simulink subsystem "Accelerometer"  (R2024b)
settings: Solver=VariableStepAuto  StartTime=0.0  StopTime=10.0  RelTol=1e-3
values from neighbouring files (symbols this model uses):
  g = 9.81    [Plant_balrob_params.m]
  ms22g = 1/g    (= 0.101936799185)    [Plant_balrob_params.m]
  Ts = 1e-2    (= 0.01)    [Plant_balrob_params.m]
undefined symbols (not defined in the file or in its folder): sens, wheel
settings Model: Creator=federico  LastModifiedBy=federico

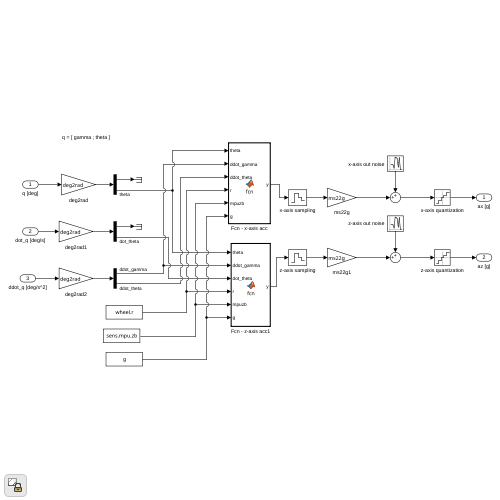
[thumbnail: Simulink's stored preview of the top-level diagram]
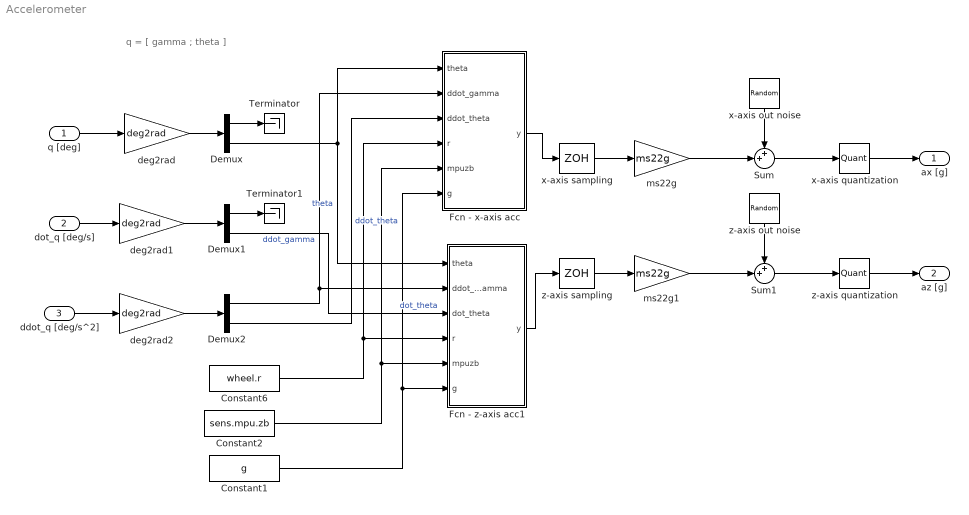
== system Accelerometer ==
  note: q = [ gamma ; theta ]
  q [deg] : Inport
  dot_q [deg/s] : Inport  Port=2
  ddot_q [deg/s^2] : Inport  Port=3
  Constant1 : Constant  Value=g
  Constant2 : Constant  Value=sens.mpu.zb
  Constant6 : Constant  Value=wheel.r
  Demux : Demux  Outputs=2
  Demux1 : Demux  Outputs=2
  Demux2 : Demux  Outputs=2
  Fcn - x-axis acc : MATLAB Function  TreatAsAtomicUnit=on
  Fcn - z-axis acc1 : MATLAB Function  TreatAsAtomicUnit=on
  Sum : Sum  Inputs=++|
  Sum1 : Sum  Inputs=++|
  Terminator : Terminator
  Terminator1 : Terminator
  deg2rad : Gain  Gain=deg2rad
  deg2rad1 : Gain  Gain=deg2rad
  deg2rad2 : Gain  Gain=deg2rad
  ms22g : Gain  Gain=ms22g
  ms22g1 : Gain  Gain=ms22g
  x-axis out noise : RandomNumber  Variance=sens.mpu.acc.noisevar  SampleTime=Ts
  x-axis quantization : Quantizer  QuantizationInterval=sens.mpu.acc.LSB2g
  x-axis sampling : ZeroOrderHold  SampleTime=Ts
  z-axis out noise : RandomNumber  Variance=sens.mpu.acc.noisevar  SampleTime=Ts
  z-axis quantization : Quantizer  QuantizationInterval=sens.mpu.acc.LSB2g
  z-axis sampling : ZeroOrderHold  SampleTime=Ts
  ax [g] : Outport
  az [g] : Outport  Port=2
  wires:
  q [deg]/1 -> deg2rad/1
  dot_q [deg/s]/1 -> deg2rad1/1
  ddot_q [deg/s^2]/1 -> deg2rad2/1
  Fcn - x-axis acc/1(y) -> x-axis sampling/1
  Fcn - z-axis acc1/1(y) -> z-axis sampling/1
  x-axis sampling/1 -> ms22g/1
  z-axis sampling/1 -> ms22g1/1
  x-axis out noise/1 -> Sum/1
  ms22g/1 -> Sum/2
  ms22g1/1 -> Sum1/2
  z-axis out noise/1 -> Sum1/1
  Sum/1 -> x-axis quantization/1
  Sum1/1 -> z-axis quantization/1
  x-axis quantization/1 -> ax [g]/1
  z-axis quantization/1 -> az [g]/1
  deg2rad/1 -> Demux/1
  deg2rad1/1 -> Demux1/1
  deg2rad2/1 -> Demux2/1
  Demux/2 -> Fcn - z-axis acc1/1(theta), Fcn - x-axis acc/1(theta)  "theta"
  Demux2/1 -> Fcn - x-axis acc/2(ddot_gamma), Fcn - z-axis acc1/2(ddot_gamma)  "ddot_gamma"
  Demux1/2 -> Fcn - z-axis acc1/3(dot_theta)  "dot_theta"
  Demux2/2 -> Fcn - x-axis acc/3(ddot_theta)  "ddot_theta"
  Demux/1 -> Terminator/1
  Demux1/1 -> Terminator1/1
  Constant6/1 -> Fcn - z-axis acc1/4(r), Fcn - x-axis acc/4(r)
  Constant2/1 -> Fcn - x-axis acc/5(mpuzb), Fcn - z-axis acc1/5(mpuzb)
  Constant1/1 -> Fcn - x-axis acc/6(g), Fcn - z-axis acc1/6(g)

== matlab function Accelerometer/Fcn - x-axis acc ==
  data: theta input; y output; ddot_gamma input; ddot_theta input; r input; mpuzb input; g input
function y = fcn(theta,ddot_gamma,ddot_theta,r,mpuzb,g)

y = r*ddot_gamma*cos(theta) + mpuzb*ddot_theta + g*sin(theta);

== matlab function Accelerometer/Fcn - z-axis acc1 ==
  data: theta input; y output; ddot_gamma input; dot_theta input; r input; mpuzb input; g input
function y = fcn(theta,ddot_gamma,dot_theta,r,mpuzb,g)

y = r*ddot_gamma*sin(theta) - mpuzb*(dot_theta^2) - g*cos(theta);
